simulink model "mm_autograde_M1a_2025a"  (R2025a)
settings: Solver=FixedStepAuto  StartTime=0.0  StopTime=30  FixedStep=0.005  RelTol=1e-3
libraries: mmuct_lib x2
settings Model: PacingRate=2  Creator=nicolls  LastModifiedBy=nicolls
settings RTWCC: GenCodeOnly=on

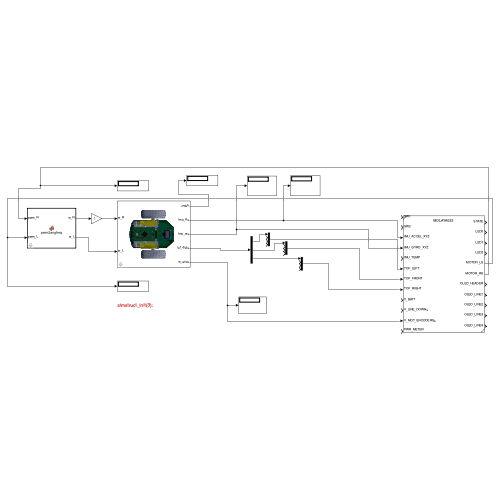
[thumbnail: Simulink's stored preview of the top-level diagram]
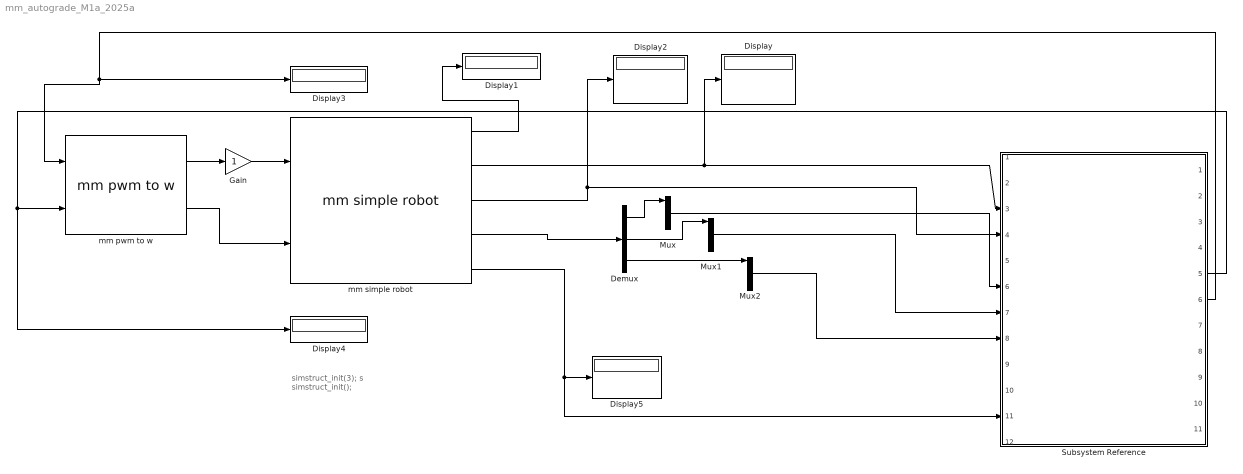
== system mm_autograde_M1a_2025a ==
  note: simstruct_init(3);
      | s
      | simstruct_init();
  Demux : Demux  Outputs=3
  Display{,1..5} (6 alike) : Display
  Gain : Gain
  Mux : Mux
  Mux1 : Mux
  Mux2 : Mux
  Subsystem Reference : Subsystem  ReferencedSubsystem=MDLAYA022
  mm pwm to w : mmuct_lib/mm pwm to w  deadb=0  maxw=2*pi  motd=0
  mm simple robot : mmuct_lib/mm simple robot  simstruct=simstruct  x0=0.3  y0=0.75  theta0=0
      settings: SourceProductName=UCT EEE Micromouse
  wires:
  Demux/1 -> Mux/1
  Demux/2 -> Mux1/1
  Demux/3 -> Mux2/1
  Subsystem Reference/6 -> Display3/1, mm pwm to w/1
  mm simple robot/3 -> Display2/1, Subsystem Reference/4
  mm simple robot/1 -> Display1/1
  mm simple robot/5 -> Subsystem Reference/11, Display5/1
  mm pwm to w/2 -> mm simple robot/2
  mm pwm to w/1 -> Gain/1
  Mux2/1 -> Subsystem Reference/8
  Mux1/1 -> Subsystem Reference/7
  Mux/1 -> Subsystem Reference/6
  mm simple robot/2 -> Subsystem Reference/3, Display/1
  Subsystem Reference/5 -> mm pwm to w/2, Display4/1
  mm simple robot/4 -> Demux/1
  Gain/1 -> mm simple robot/1
